simulink model "P_2_2_ramp_error"  (R2021a)
settings: Solver=VariableStepAuto  StartTime=0.0  StopTime=10.0  RelTol=1e-3
settings Model: Creator=alamg  LastModifiedBy=alamg

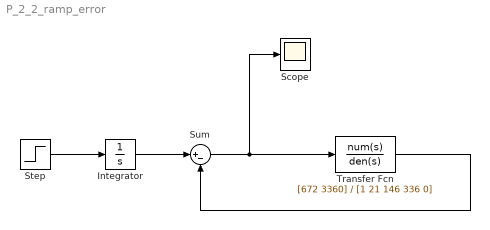
== system P_2_2_ramp_error ==
  Integrator : Integrator
  Scope : Scope
  Step : Step  SampleTime=0
  Sum : Sum  Inputs=|+-
  Transfer Fcn : TransferFcn  Numerator=[672 3360]  Denominator=[1 21 146 336 0]
  wires:
  Sum/1 -> Transfer Fcn/1, Scope/1
  Transfer Fcn/1 -> Sum/2
  Integrator/1 -> Sum/1
  Step/1 -> Integrator/1
